simulink model "ammoniawithfuzzynew"  (R2024a)
settings: Solver=VariableStepAuto  StartTime=0.0  StopTime=10.0  RelTol=1e-3
libraries: neural x83
(part 3 of 3)

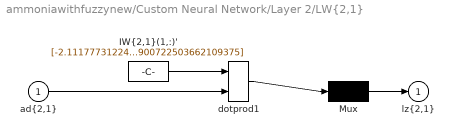
== system ammoniawithfuzzynew/Custom Neural Network/Layer 2/LW{2,1} ==
  "ad{2,1}" : Inport  PortDimensions=80
      mask Display: e = 0.06;c1 = [120 230 180]/255;c2 = ([120 230 180]+0)/(256+128);c3 = ([120 230 180]+128)/(256+128);patch([0 1 1 0],[0 0 1 1],c1);patch([0 1 1 1-e 1-e 0+e],[0 0 1 1-e 0+e 0+e],c2);patch([0 0 1 1-e 0+e 0+e],[0 1 1 1-e 1-e 0+e],c3);plot([0 1 1 0 0],[0 0 1 1 0]);
  "IW{2,1}(1,:)'" : Constant  Value=[-2.11177731224954445821140325278975069522857666015625;-0.73618978739356777385438590499688871204853057861328125;-10.9333532319803925503265418228693306446075439453125;25.6240715382595141136334859766066074371337890625;-0.359303787316451295197339277365244925022125244140625;-1.902756361631043002802243790938518941402435302734375;2.9990384434563690518871226231567561626434326171875;-0.264109487992577829373885833774693310260772705078125;-4.3420308426402325352455591200850903987884521484375;-5.6268298257380617855005766614340245723724365234375;-1.7147790939301634782765404452220536768436431884765625;-0.0940020131986837037540993833317770622670650482177734375;10.55258146429736854088332620449364185333251953125;-5.66914774806321286604315901058726012706756591796875;-12.42594778762239826619406812824308872222900390625;0.64728694842289946631552766120876185595989227294921875;-11.33510419906308896997870760969817638397216796875;-21.769014869679377710554035729728639125823974609375;0.07998180650366561172948109970093355514109134674072265625;-12.5373255248394972483083620318211615085601806640625;-1.6290045186658208553609483715263195335865020751953125;-2.67750494726989440863462732522748410701751708984375;-14.3315811599069267145978301414288580417633056640625;30.78412284771273021988235996104776859283447265625;-45.24136945192896774869950604625046253204345703125;5.35331405463233078734219816396944224834442138671875;22.169746134168281770371322636492550373077392578125;-0.50010399452827625221829066504142247140407562255859375;60.83781897863726584319010726176202297210693359375;58.00855435445379981729274732060730457305908203125;4.80152300375007801136462148861028254032135009765625;-17.8865889792910053301966399885714054107666015625;-14.084987624852391974172860500402748584747314453125;9.6228212845298219946243989397771656513214111328125;0.5373788042422622535099208107567392289638519287109375;3.372436333412593523206624013255350291728973388671875;28.87199356053539389677098370157182216644287109375;33.62214825369816395550515153445303440093994140625;-10.1838282274581377606637033750303089618682861328125;-28.1826494822140602991566993296146392822265625;-2.034796738529800474992725867195986211299896240234375;-16.95736201593782510599339730106294155120849609375;5.931296092938726616239364375360310077667236328125;-8.019389496491566404756667907349765300750732421875;44.56246820602209623984890640713274478912353515625;-5.24373498895773071382109264959581196308135986328125;-15.902014672658435046059821615926921367645263671875;18.334504876471470424803555943071842193603515625;24.576282066824891359146931790746748447418212890625;22.324697704138511511473552673123776912689208984375;-3.8104805038723466026340247481130063533782958984375;-0.96629366896612933768295761183253489434719085693359375;-11.4295768071869385806849095388315618038177490234375;-2.42446893216086056810354421031661331653594970703125;-16.8735121905508407280649407766759395599365234375;-4.0650680459009667089276263141073286533355712890625;-1.885713566463277590656844040495343506336212158203125;0.7286390877077721928145592755754478275775909423828125;8.73909056972322417777832015417516231536865234375;3.66457222923845815643062451272271573543548583984375;9.4759688163237996150201070122420787811279296875;-10.8168039955439798660563610610552132129669189453125;9.2849259524084839512170219677500426769256591796875;1.9230908156331538716443674275069497525691986083984375;-4.3505452706194365219971587066538631916046142578125;-19.652315103726184730703607783652842044830322265625;-13.167210137409742998215733678080141544342041015625;8.061273658777640349626381066627800464630126953125;-8.7859206201897901422626091516576707363128662109375;-1.0136823983580445229790711891837418079376220703125;0.44835419237636708889027659097337163984775543212890625;-1.03369325759015051602318635559640824794769287109375;-4.27449462012562975132823339663445949554443359375;-6.2008518846355737963449428207240998744964599609375;5.97625416509155460431657047593034803867340087890625;0.8539268154268666588535552364191971719264984130859375;-17.6424942019448423025096417404711246490478515625;-5.2732846463882712129134233691729605197906494140625;-2.37146674643834121098961986717768013477325439453125;-15.3844708913007703898756517446599900722503662109375]
      mask Display: e = 0.06;c1 = [120 150 230]/255;c2 = ([120 150 230]+0)/383;c3 = ([120 150 230]+128)/383;patch([0 1 1 0],[0 0 1 1],c1);patch([0 1 1 1-e 1-e 0+e],[0 0 1 1-e 0+e 0+e],c2);patch([0 0 1 1-e 0+e 0+e],[0 1 1 1-e 1-e 0+e],c3);plot([0 1 1 0 0],[0 0 1 1 0]);disp('weights');
  Mux : Mux  Inputs=1
      mask Display: e = 0.06;c1 = [120 150 230]/255;c2 = ([120 150 230]+0)/383;c3 = ([120 150 230]+128)/383;patch([0 1 1 0],[0 0 1 1],c1);patch([0 1 1 1-e 1-e 0+e],[0 0 1 1-e 0+e 0+e],c2);patch([0 0 1 1-e 0+e 0+e],[0 1 1 1-e 1-e 0+e],c3);plot([0 1 1 0 0],[0 0 1 1 0]);disp('Mux');
  dotprod1 : neural/Weight Functions/dotprod
  "lz{2,1}" : Outport
      mask Display: e = 0.06;c1 = [120 230 180]/255;c2 = ([120 230 180]+0)/(256+128);c3 = ([120 230 180]+128)/(256+128);patch([0 1 1 0],[0 0 1 1],c1);patch([0 1 1 1-e 1-e 0+e],[0 0 1 1-e 0+e 0+e],c2);patch([0 0 1 1-e 0+e 0+e],[0 1 1 1-e 1-e 0+e],c3);plot([0 1 1 0 0],[0 0 1 1 0]);
  wires:
  "IW{2,1}(1,:)'"/1 -> dotprod1/1
  "ad{2,1}"/1 -> dotprod1/2
  dotprod1/1 -> Mux/1
  Mux/1 -> "lz{2,1}"/1

== matlab function ammoniawithfuzzynew/MATLAB Function1 ==
  data: Q input; Q output; Q_control input; T_delayed input
function Q = heat_power_dynamics(Q, Q_control, T_delayed)
    % Parameters
    alpha = 0.1;
    T_ambient = 300;
    dt = 0.1;
    
    % Calculate the rate of change of heat power
    dQ = Q_control - alpha * (T_delayed - T_ambient);
    
    % Update the heat power value
    Q = Q + dQ * dt;
end

== matlab function ammoniawithfuzzynew/MATLAB Function ==
  settings: updateMethod=DISCRETE  sampleTime=0.1
  data: temperature input; concentration input; heatPower input; controlSignal output size=[1 1]
function controlSignal = evaluateFIS(temperature, concentration, heatPower)
    % Preinitialize the output variable
    controlSignal = 0; % Initial value, preinitialized as a scalar double
    
    % Use coder.extrinsic to declare evalfis as an external function
    coder.extrinsic('evalfis');
    
    % Load the pre-processed FIS data
    persistent fisCodeGenData;
    if isempty(fisCodeGenData)
        fisData = load('AmmoniaControlFIS_CG.mat');
        fisCodeGenData = fisData.fisCodeGenData;
    end
    
    % Create an input matrix
    inputs = [temperature, concentration, heatPower];
    
    % Evaluate the FIS using evalfis
    controlSignal = evalfis(fisCodeGenData, inputs);
    
    % Ensure controlSignal is a scalar double
    controlSignal = double(controlSignal);
end

== matlab function ammoniawithfuzzynew/MATLAB Function2 ==
  data: T input; T output; Q_delayed input; Q_out input
function T = temperature_dynamics(T, Q_delayed, Q_out)
    % Parameters
    m = 10;
    C_p = 4.18;
    Delta_H = -92000; % in J/mol
    r = 0.1;
    rho = 0.001;
    dt = 0.1;
    
    % Calculate the rate of change of temperature
    dT = (Q_delayed - Q_out) / (m * C_p) + (Delta_H * r) / (rho * C_p);
    
    % Update the temperature value
    T = T + dT * dt;
end

== matlab function ammoniawithfuzzynew/MATLAB Function3 ==
  data: C_NH3 input; C_NH3 output; T input
function C_NH3 = concentration_dynamics(C_NH3, T)
    % Parameters
    F_in = 1;
    C_in = 0.05;
    F_out = 1;
    V = 1;
    dt = 0.1;
    
    % Calculate the reaction rate based on temperature (T) and ammonia concentration (C_NH3)
    if T > 300 && C_NH3 > 0.5
        r = 0.1 * T * C_NH3;
    else
        r = 0.05 * T;
    end
    
    % Calculate the rate of change of ammonia concentration
    dC_NH3 = -r + (F_in * C_in - F_out * C_NH3) / V;
    
    % Update the concentration value
    C_NH3 = C_NH3 + dC_NH3 * dt;
end
